simulink model "LF_AC29bus_HVDCdemo_V2_1"  (R2019b)
settings: Solver=FixedStepDiscrete  StartTime=0.0  StopTime=fix(6/Ts)*Ts  FixedStep=Ts  RelTol=1e-3
InitFcn:
  | Ts_avg=150e-6;
  | Ts=50e-6;
  | 
  | %Tc_stab = 1/60/5;
  | %Tc_stab = 2/60;
  | Tc_stab = Ts;
  | 
  | 
  | Ts_avg=150e-6;
  | 
  | Ts=50e-6;
  | 
  | % Rectifier AC side :
  | VLL_nom_R = 735e3; % V
  | Fnom_R = 60;           % Hz
  | 
  | % Inverter AC side :
  | VLL_nom_I = 735e3; % V
  | Fnom_I = 60;           % Hz
  | 
  | % DC :
  | Vdc_nom = 500e3;   % V
  | Idc_nom  = 2000;     % A
undefined symbols (not defined in the file): D1, D11, Delta, test_alpha
libraries: powerlib x223, powerlib_meascontrol x57, simulink x22, sps_avr x7
(part 4 of 10)

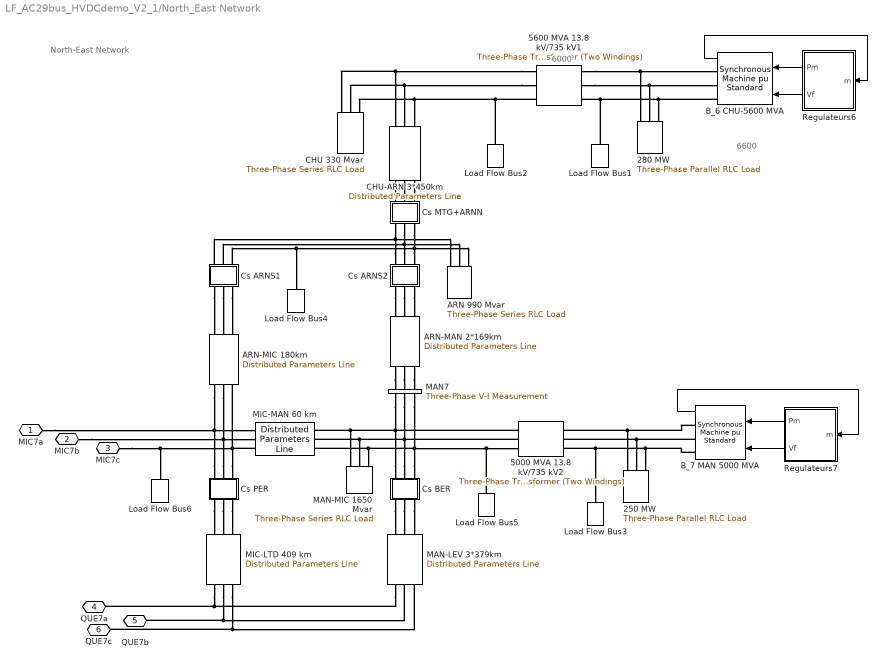
== system LF_AC29bus_HVDCdemo_V2_1/North_East Network ==
  note: 6600
  note: 6000
  note: North-East Network
  250 MW : powerlib/Elements/Three-Phase Parallel RLC Load  LConnTagsString=A|B|C  Configuration=Y (grounded)  NominalVoltage=(13800)*1  Vabc=[1e3 1e3 1e3]  Vabcp=[1e3 1e3 1e3]  NominalFrequency=60  UnbalancedPower=off  ActivePower=250000000  InductivePower=0  CapacitivePower=0  Pabc=[10e3 9e3 11e3]  QLabc=[100 90 110]  QCabc=[100 90 110]  Pabcp=[10e3 9e3 11e3]  QLabcp=[100 90 110]  QCabcp=[100 90 110]  Measurements=None  LoadType=constant PQ
      settings: SourceProductName=Simscape Electrical
  280 MW : powerlib/Elements/Three-Phase Parallel RLC Load  LConnTagsString=A|B|C  Configuration=Y (grounded)  NominalVoltage=(13800)*1  Vabc=[1e3 1e3 1e3]  Vabcp=[1e3 1e3 1e3]  NominalFrequency=60  UnbalancedPower=off  ActivePower=280000000  InductivePower=0  CapacitivePower=0  Pabc=[10e3 9e3 11e3]  QLabc=[100 90 110]  QCabc=[100 90 110]  Pabcp=[10e3 9e3 11e3]  QLabcp=[100 90 110]  QCabcp=[100 90 110]  Measurements=None  LoadType=constant PQ
      settings: SourceProductName=Simscape Electrical
  5000 MVA 13.8 kV/735 kV2 : powerlib/Elements/Three-Phase Transformer (Two Windings)  Winding1Connection=Delta (D1)  Winding2Connection=Yg  CoreType=Three single-phase transformers  SetSaturation=off  Hysteresis=off  DataFile='basic_model'  SetInitialFlux=off  Measurements=None  UNITS=pu  NominalPower=[ 5000e6 60 ]  Winding1="[ 13.8e3 0.002  0.0]"  Winding2=[ 735e3 0.002 0.12]  Rm=500  Lm=500  L0=0.5  Saturation="[ 0,0  ;  0.005,1.2  ;  1.0,1.4 ]"  InitialFluxes=[ 0.8 , -0.8 , 0.7 ]  BreakLoop=off  DiscreteSolver=Trapezoidal iterative  DataType=off  TransfoNumber=0
      settings: SourceProductName=Simscape Electrical
  5600 MVA 13.8 kV/735 kV1 : powerlib/Elements/Three-Phase Transformer (Two Windings)  Winding1Connection=Delta (D1)  Winding2Connection=Yg  CoreType=Three single-phase transformers  SetSaturation=off  Hysteresis=off  DataFile='basic_model'  SetInitialFlux=off  Measurements=None  UNITS=pu  NominalPower=[ 5600e6 60 ]  Winding1="[ 13.8e3 0.002  0.0]"  Winding2=[ 735e3 0.002 0.12]  Rm=500  Lm=500  L0=0.5  Saturation="[ 0,0  ;  0.005,1.2  ;  1.0,1.4 ]"  InitialFluxes=[ 0.8 , -0.8 , 0.7 ]  BreakLoop=off  DiscreteSolver=Trapezoidal iterative  DataType=off  TransfoNumber=0
      settings: SourceProductName=Simscape Electrical
  ARN 990 Mvar : powerlib/Elements/Three-Phase Series RLC Load  LConnTagsString=A|B|C  Configuration=Y (grounded)  NominalVoltage=735e3  Vabc=[1e3 1e3 1e3]  Vabcp=[1e3 1e3 1e3]  NominalFrequency=60  UnbalancedPower=off  ActivePower=3300000  InductivePower=990e6  CapacitivePower=0  Pabc=[10e3 9e3 11e3]  QLabc=[100 90 110]  QCabc=[100 90 110]  Pabcp=[10e3 9e3 11e3]  QLabcp=[100 90 110]  QCabcp=[100 90 110]  Measurements=None  LoadType=constant Z
      settings: SourceProductName=Simscape Electrical
  ARN-MAN 2*169km : powerlib/Elements/Distributed Parameters Line  Phases=3  Frequency=60  Resistance="[0.01273  0.3864]/2"  Inductance="[0.9337e-3  4.1264e-3]/2"  Capacitance=[12.74e-9 7.751e-9]*2  Length=169  x1=[-0.001 1.77895403371725e-09 0 0;-0.00095 1.78335877274119e-09 0 0;-0.0009 1.78712989288485e-09 0 0;-0.00085 1.79026605428719e-09 0 0;-0.0008 1.79276614268501e-09 0 0;-0.00075 1.7946292698088e-09 0 0;-0.0007 1.79585477369837e-09 0 0;-0.00065 1.79644221893802e-09 0 0;-0.0006 1.79639139681125e-09 447147.457758488 -644889.053445503;-0.00055 1.79570232537492e-09 459223.19701965 -636346.501015419;-0.0005 1.79437524945284e-09 471135.776465557 -627577.857703564;-0.00045 1.79241064054876e-09 482880.963613455 -618586.238967152;-0.0004 1.78980919667886e-09 494454.585454275 -609374.839485507;-0.00035 1.78657184212377e-09 505852.529935287 -599946.932025003;-0.0003 1.78269972710015e-09 517070.747421089 -590305.866276268;-0.00025 1.77819422735202e-09 528105.252132427 -580455.067664057;-0.0002 1.773056943662e-09 538952.123562317 -570398.03613021;-0.00015 1.76728970128251e-09 549607.507868989 -560138.344890143;-0.0001 1.76089454928731e-09 560067.619245137 -549679.639163302;-5e-05 1.75387375984347e-09 570328.741262995 -539025.63487803]  x2=[-0.001 3.40571061718068e-09 0 0;-0.00095 3.40987138108151e-09 0 0;-0.0009 3.41282063391716e-09 0 0;-0.00085 3.41455732783211e-09 0 0;-0.0008 3.41508084578731e-09 0 0;-0.00075 3.41439100177931e-09 0 0;-0.0007 3.41248804090641e-09 0 0;-0.00065 3.40937263928153e-09 0 0;-0.0006 3.40504590379205e-09 338825.124939883 -670601.319593136;-0.00055 3.39950937170648e-09 351404.740366806 -664095.897634329;-0.0005 3.39276501012831e-09 363859.503362732 -657354.525565264;-0.00045 3.38481521529709e-09 376184.988809673 -650379.598563337;-0.0004 3.37566281173707e-09 388376.817521339 -643173.5947869;-0.00035 3.36531105125365e-09 400430.657799042 -635739.074494781;-0.0003 3.35376361177806e-09 412342.226970727 -628078.679136641;-0.00025 3.34102459606054e-09 424107.292912585 -620195.130414475;-0.0002 3.32709853021272e-09 435721.675552709 -612091.229315605;-0.00015 3.31199036209949e-09 447181.248356249 -603769.855117503;-0.0001 3.29570545958104e-09 458481.939791554 -595233.9643648;-5e-05 3.27824960860569e-09 469619.734776766 -586486.589818835]  x3=[-0.001 4.69891861565071e-12 0 0;-0.00095 4.9976044278027e-12 0 0;-0.0009 5.29451461489816e-12 0 0;-0.00085 5.58954368616142e-12 0 0;-0.0008 5.88258681916825e-12 0 0;-0.00075 6.17353989708886e-12 0 0;-0.0007 6.46229954568008e-12 0 0;-0.00065 6.74876317001371e-12 0 0;-0.0006 7.03282899092808e-12 1762.60496260231 -1477.81528810955;-0.00055 7.31439608118961e-12 1790.14624540764 -1444.33079403529;-0.0005 7.59336440135186e-12 1817.05149777597 -1410.33313610726;-0.00045 7.869634835299e-12 1843.31116039924 -1375.83439353143;-0.0004 8.14310922546136e-12 1868.91590334437 -1340.84682354679;-0.00035 8.41369040769029e-12 1893.85662936811 -1305.38285707033;-0.0003 8.68128224578015e-12 1918.12447714925 -1269.45509428049;-0.00025 8.94578966562503e-12 1941.71082443704 -1233.07630014032;-0.0002 9.20711868899815e-12 1964.60729111459 -1196.25939986214;-0.00015 9.46517646694184e-12 1986.80574217631 -1159.01747431533;-0.0001 9.71987131275639e-12 2008.29829061826 -1121.36375537869;-5e-05 9.97111273457583e-12 2029.07730024029 -1083.31162123926]  x4=[-0.001 5.93929013944843e-12 0 0;-0.00095 5.74454886917117e-12 0 0;-0.0009 5.54776658803405e-12 0 0;-0.00085 5.34901321184454e-12 0 0;-0.0008 5.14835935673082e-12 0 0;-0.00075 4.94587631405218e-12 0 0;-0.0007 4.74163602506952e-12 0 0;-0.00065 4.53571105538502e-12 0 0;-0.0006 4.32817456915987e-12 2941.48430270319 -8820.70411387501;-0.00055 4.11910030311941e-12 3107.21872626171 -8763.69488470381;-0.0005 3.90856254035483e-12 3271.84916980218 -8703.57195646944;-0.00045 3.69663608393074e-12 3435.31714091192 -8640.35669056202;-0.0004 3.483396230308e-12 3597.56456019916 -8574.07154706452;-0.00035 3.26891874259124e-12 3758.53378192839 -8504.7400767728;-0.0003 3.05327982361058e-12 3918.1676145016 -8432.38691282813;-0.00025 2.83655608884714e-12 4076.4093407782 -8357.03776196514;-0.0002 2.61882453921192e-12 4233.20273822633 -8278.71939537834;-0.00015 2.40016253368777e-12 4388.49209889845 -8197.45963921046;-0.0001 2.18064776184406e-12 4542.22224922416 -8113.28736466595;-5e-05 1.96035821623397e-12 4694.33856961305 -8026.23247775314]  x5=0.000955765248222805  V1=ones(3,3)  V2=ones(3,3)  I1=ones(3,3)  I2=ones(3,3)  nHarmo=1  Measurements=None
      settings: AttributesFormatString=\n  SourceProductName=Simscape Electrical
  ARN-MIC 180km : powerlib/Elements/Distributed Parameters Line  Phases=3  Frequency=60  Resistance="[0.01273  0.3864]"  Inductance="[0.9337e-3  4.1264e-3]"  Capacitance=[12.74e-9 7.751e-9]  Length=180  x1=[-0.00105 1.65528202570484e-09 337720.166187843 -692555.258770577;-0.001 1.65999997031716e-09 350713.785460204 -686066.768257753;-0.00095 1.66412812484431e-09 363582.797794555 -679334.521488954;-0.0009 1.66766502257264e-09 376322.630892093 -672360.910399402;-0.00085 1.67060940685924e-09 388928.758350779 -665148.412679911;-0.0008 1.67296023157838e-09 401396.701273553 -657699.590896577;-0.00075 1.67471666149325e-09 413722.029859663 -650017.091580312;-0.0007 1.67587807255264e-09 425900.364978549 -642103.644286542;-0.00065 1.67644405211275e-09 437927.379725734 -633962.060625409;-0.0006 1.67641439908373e-09 449798.800960145 -625595.233262821;-0.00055 1.67578912400116e-09 461510.410822345 -617006.1348927;-0.0005 1.6745684490223e-09 473058.048233116 -608197.8171808;-0.00045 1.67275280784716e-09 484437.610371872 -599173.40968046;-0.0004 1.6703428455644e-09 495645.054134369 -589936.118720696;-0.00035 1.66733941842215e-09 506676.397569205 -580489.226267001;-0.0003 1.66374359352376e-09 517527.721292583 -570836.088755282;-0.00025 1.6595566484487e-09 528195.169880856 -560980.135899331;-0.0002 1.65478007079863e-09 538674.953240334 -550924.869472268;-0.00015 1.64941555766883e-09 548963.34795389 -540673.862062376;-0.0001 1.64346501504528e-09 559056.698603872 -530230.755803775;-5e-05 1.63693055712744e-09 568951.419070854 -519599.261082393]  x2=[-0.00105 2.20757216589407e-09 202405.879598002 -745458.867777492;-0.001 2.20435426546261e-09 216420.682546405 -741511.432952835;-0.00095 2.20035316845693e-09 230358.592256812 -737300.542646845;-0.0009 2.19557029644773e-09 244214.65665627 -732827.692968796;-0.00085 2.19000734876668e-09 257983.952751074 -728094.47310088;-0.0008 2.18366630190258e-09 271661.588375888 -723102.56473358;-0.00075 2.17654940879921e-09 285242.7039319 -717853.741468168;-0.0007 2.16865919805479e-09 298722.474113422 -712349.868186557;-0.00065 2.15999847302362e-09 312096.109622293 -706592.900388718;-0.0006 2.15057031082007e-09 325358.858869498 -700584.883497896;-0.00055 2.14037806122529e-09 338506.009663382 -694327.952133885;-0.0005 2.12942534549702e-09 351532.890883869 -687824.329354606;-0.00045 2.117716055083e-09 364434.874142089 -681076.325866263;-0.0004 2.10525435023836e-09 377207.375424827 -674086.339202365;-0.00035 2.0920446585475e-09 389845.856723194 -666856.852871891;-0.0003 2.07809167335098e-09 402345.827644964 -659390.435476908;-0.00025 2.06340035207799e-09 414702.847009989 -651689.739799966;-0.0002 2.04797591448504e-09 426912.524428128 -643757.501861571;-0.00015 2.03182384080135e-09 438970.521859132 -635596.539948092;-0.0001 2.01494986978179e-09 450872.555153929 -627209.753610437;-5e-05 1.99735999666791e-09 462614.395576763 -618600.122633857]  x3=[-0.00105 4.80507864505899e-12 25.4663662601597 -574.53320615078;-0.001 4.83653768049388e-12 36.2908676891206 -573.951344402014;-0.00095 4.86627831712063e-12 47.1024751455949 -573.165560473519;-0.0009 4.89428998823267e-12 57.8973473169339 -572.176133550583;-0.00085 4.92056274141663e-12 68.6716488364564 -570.983415171881;-0.0008 4.94508724208841e-12 79.4215516461353 -569.587829104573;-0.00075 4.96785477680969e-12 90.1432363566896 -567.989871193744;-0.0007 4.98885725638379e-12 100.832893604594 -566.19010918623;-0.00065 5.00808721872974e-12 111.486725405528 -564.189182528904;-0.0006 5.02553783153347e-12 122.100946503783 -561.987802141478;-0.00055 5.04120289467534e-12 132.671785717143 -559.586750163923;-0.0005 5.05507684243302e-12 143.195487276771 -556.986879678573;-0.00045 5.06715474545893e-12 153.668312161611 -554.189114407032;-0.0004 5.07743231253163e-12 164.08653942685 -551.19444838198;-0.00035 5.08590589208049e-12 174.446467525947 -548.003945593994;-0.0003 5.09257247348302e-12 184.744415625781 -544.618739613524;-0.00025 5.09742968813462e-12 194.976724914425 -541.040033188136;-0.0002 5.10047581029003e-12 205.139759901111 -537.269097815182;-0.00015 5.10170975767657e-12 215.229909707902 -533.307273290045;-0.0001 5.10113109187859e-12 225.243589352616 -529.155967230113;-5e-05 5.09874001849331e-12 235.177241022557 -524.816654574663]  x4=[-0.00105 7.01566942822821e-13 1335.19730340444 -4937.0942549236;-0.001 6.80396887210245e-13 1428.01688045782 -4911.05082799012;-0.00095 6.58985089823434e-13 1520.32908991326 -4883.262528082;-0.0009 6.37339158172044e-13 1612.10113368227 -4853.73922824988;-0.00085 6.15466782952521e-13 1703.3004055947 -4822.49141798161;-0.0008 5.93375735315632e-13 1793.89450298348 -4789.5301994754;-0.00075 5.71073864105415e-13 1883.8512381972 -4754.86728369523;-0.0007 5.48569093070516e-13 1973.13865003616 -4718.51498621003;-0.00065 5.25869418048926e-13 2061.7250151081 -4680.48622281798;-0.0006 5.02982904127093e-13 2149.57885909932 -4640.79450495766;-0.00055 4.79917682774435e-13 2236.66896795737 -4599.45393490742;-0.0005 4.56681948954273e-13 2322.96439898127 -4556.47920077495;-0.00045 4.33283958212192e-13 2408.43449181528 -4511.88557127866;-0.0004 4.09732023742891e-13 2493.0488793424 -4465.68889032277;-0.00035 3.86034513436542e-13 2576.77749847363 -4417.90557136805;-0.0003 3.62199846905717e-13 2659.59060082928 -4368.5525916002;-0.00025 3.38236492493944e-13 2741.45876330842 -4317.64748589794;-0.0002 3.14152964266941e-13 2822.35289854272 -4265.20834060292;-0.00015 2.89957818987611e-13 2902.24426523115 -4211.25378709378;-0.0001 2.65659653075862e-13 2981.10447835151 -4155.80299516647;-5e-05 2.41267099554346e-13 3058.9055192456 -4098.87566622332]  x5=0.00101797482059234  V1=ones(3,3)  V2=ones(3,3)  I1=ones(3,3)  I2=ones(3,3)  nHarmo=1  Measurements=None
      settings: AttributesFormatString=\n  SourceProductName=Simscape Electrical
  "B_6 CHU-5600 MVA " : powerlib/Machines/Synchronous Machine pu Standard  PresetModel=No  MechanicalLoad=Mechanical power Pm  ShowDetailedParameters=on  RotorType=Salient-pole  Units=per unit standard parameters  MeasurementBus=off  NominalParameters="[ 5600E6  13800   60 ]"  Reactances1=[ 31 32 33 34 35 36 37 ]  Reactances2=[ 1.305, 0.296, 0.252, 0.474, 0.243, 0.18 ]  dAxisTimeConstants=Short-circuit  qAxisTimeConstants=Open-circuit  TimeConstants1=[]  TimeConstants2=[]  TimeConstants3=[]  TimeConstants4=[]  TimeConstants5=[ 1.01, 0.053, 0.1 ]  TimeConstants6=[]  TimeConstants7=[]  TimeConstants8=[]  StatorResistance=2.8544e-3  Mechanical="[ 4.0 0  32]"  PolePairs=32  InitialConditions=[0 -59.3146 0.896045 0.896045 0.896045 11.8671 -108.133 131.867 1.2956]  SetSaturation=off  Saturation=[0.6404,0.7127,0.8441,0.9214,0.9956,1.082,1.19,1.316,1.457;0.7,0.7698,0.8872,0.9466,0.9969,1.046,1.1,1.151,1.201]  LoadFlowParameters=[1 5000000000 0 0 0]  TsPowergui=0  TsBlock=-1  IterativeModel=Trapezoidal non iterative  IterativeDiscreteModel=Trapezoidal non iterative  BusType=PV  Pref=5000000000  Qref=0  Qmin=-Inf  Qmax=Inf  PLF=0  QLF=0
      settings: AttributesFormatString=\n\n  SourceProductName=Simscape Electrical
  B_7 MAN 5000 MVA : powerlib/Machines/Synchronous Machine pu Standard  PresetModel=No  MechanicalLoad=Mechanical power Pm  ShowDetailedParameters=on  RotorType=Salient-pole  Units=per unit standard parameters  MeasurementBus=off  NominalParameters="[ 5000E6  13800   60 ]"  Reactances1=[ 31 32 33 34 35 36 37 ]  Reactances2=[ 1.305, 0.296, 0.252, 0.474, 0.243, 0.18 ]  dAxisTimeConstants=Short-circuit  qAxisTimeConstants=Open-circuit  TimeConstants1=[]  TimeConstants2=[]  TimeConstants3=[]  TimeConstants4=[]  TimeConstants5=[ 1.01, 0.053, 0.1 ]  TimeConstants6=[]  TimeConstants7=[]  TimeConstants8=[]  StatorResistance=2.8544e-3  Mechanical="[ 3.7 0  32]"  PolePairs=32  InitialConditions=[0 -78.7337 0.918283 0.918283 0.918283 -2.27692 -122.277 117.723 1.18952]  SetSaturation=off  Saturation=[0.6404,0.7127,0.8441,0.9214,0.9956,1.082,1.19,1.316,1.457;0.7,0.7698,0.8872,0.9466,0.9969,1.046,1.1,1.151,1.201]  LoadFlowParameters=[1 4500000000 0 0 0]  TsPowergui=0  TsBlock=-1  IterativeModel=Trapezoidal non iterative  IterativeDiscreteModel=Trapezoidal non iterative  BusType=PV  Pref=4500000000  Qref=0  Qmin=-Inf  Qmax=Inf  PLF=0  QLF=0
      settings: AttributesFormatString=\n\n  SourceProductName=Simscape Electrical
  CHU 330 Mvar : powerlib/Elements/Three-Phase Series RLC Load  LConnTagsString=A|B|C  Configuration=Y (grounded)  NominalVoltage=735e3  Vabc=[1e3 1e3 1e3]  Vabcp=[1e3 1e3 1e3]  NominalFrequency=60  UnbalancedPower=off  ActivePower=1100000  InductivePower=330e6  CapacitivePower=0  Pabc=[10e3 9e3 11e3]  QLabc=[100 90 110]  QCabc=[100 90 110]  Pabcp=[10e3 9e3 11e3]  QLabcp=[100 90 110]  QCabcp=[100 90 110]  Measurements=None  LoadType=constant Z
      settings: SourceProductName=Simscape Electrical
  CHU-ARN 3*450km : powerlib/Elements/Distributed Parameters Line  Phases=3  Frequency=60  Resistance="[0.01273  0.3864]/3"  Inductance="[0.9337e-3  4.1264e-3]/3"  Capacitance=[12.74e-9 7.751e-9]*3  Length=450  x1=[-0.00255 -1.47668636008146e-09 70526.907999489 -734521.053767666;-0.0025 -1.43959841142251e-09 84359.0049084098 -733061.266602517;-0.00245 -1.40199898030279e-09 98161.1294645721 -731341.026259902;-0.0024 -1.36390142562115e-09 111928.377838841 -729360.943933024;-0.00235 -1.32531928325737e-09 125655.858593425 -727121.723135704;-0.0023 -1.28626626126292e-09 139338.694419775 -724624.15945243;-0.00225 -1.24675623499054e-09 152972.023871476 -721869.140255687;-0.0022 -1.20680324216445e-09 166551.003091489 -718857.644390675;-0.00215 -1.16642147789276e-09 180070.807533156 -715590.741827537;-0.0021 -1.12562528962402e-09 193526.633674335 -712069.593281197;-0.00205 -1.08442917204968e-09 206913.70072407 -708295.449798968;-0.002 -1.04284776195414e-09 220227.252321181 -704269.652316058;-0.00195 -1.00089583301443e-09 233462.558224181 -699993.631179143;-0.0019 -9.58588290551127e-10 246614.915991903 -695468.905638173;-0.00185 -9.15940166232625e-10 259679.652654259 -690697.083306586;-0.0018 -8.72966612734418e-10 272652.126372523 -685679.859590136;-0.00175 -8.29682898355439e-10 285527.728088551 -680419.01708452;-0.0017 -7.86104401593308e-10 298301.883162364 -674916.424942028;-0.00165 -7.4224660568042e-10 310970.052997488 -669174.038207449;-0.0016 -6.98125093082829e-10 323527.736653504 -663193.897123447;-0.00155 -6.53755539963869e-10 335970.472445202 -656978.126405672;-0.0015 -6.09153710614495e-10 348293.839527803 -650528.934487864;-0.00145 -5.64335451852297e-10 360493.459467662 -643848.612737203;-0.0014 -5.19316687391205e-10 372564.997797904 -636939.534640197;-0.00135 -4.74113412183872e-10 384504.165558441 -629804.154959397;-0.0013 -4.28741686738736e-10 396306.720819817 -622445.008861226;-0.00125 -3.83217631413806e-10 407968.470190347 -614864.711015252;-0.0012 -3.37557420689171e-10 419485.270306009 -607065.954665206;-0.00115 -2.91777277420284e-10 430853.029302559 -599051.510672083;-0.0011 -2.45893467074062e-10 442067.708269356 -590824.226529673;-0.00105 -1.99922291949839e-10 453125.322684362 -582387.025352856;-0.001 -1.53880085387241e-10 464021.943829828 -573742.904839035;-0.00095 -1.07783205963022e-10 474753.700188146 -564894.93620307;-0.0009 -6.1648031678947e-11 485316.778817384 -555846.263086086;-0.00085 -1.54909541427609e-11 495707.426706 -546600.100438555;-0.0008 3.067162725567e-11 505921.952106278 -537159.73337804;-0.00075 7.68233111709838e-11 515956.725845979 -527528.516022004;-0.0007 1.22947700129642e-10 525808.182617776 -517709.870296115;-0.00065 1.69028406355873e-10 535472.822245987 -507707.284718447;-0.0006 2.15049057594176e-10 544947.210930171 -497524.313160026;-0.00055 2.60993302926296e-10 554227.982465141 -487164.57358216;-0.0005 3.06844818580638e-10 563311.839436964 -476631.746750992;-0.00045 3.52587313732015e-10 572195.554394511 -465929.574929742;-0.0004 3.98204536289709e-10 580875.970996158 -455061.860549098;-0.00035 4.43680278671758e-10 589350.005131219 -444032.464856231;-0.0003 4.88998383563431e-10 597614.646015717 -432845.306542914;-0.00025 5.34142749657847e-10 605666.957262098 -421504.360353226;-0.0002 5.79097337376693e-10 613504.077922519 -410013.655671348;-0.00015 6.2384617456901e-10 621123.223505326 -398377.275089938;-0.0001 6.68373362186019e-10 628521.686964373 -386599.352959609;-5e-05 7.12663079929983e-10 635696.839660821 -374684.073920012]  x2=[-0.00255 1.63896785414151e-09 -245055.631636569 -719265.627917785;-0.0025 1.65992719155378e-09 -231455.029793756 -723756.779042432;-0.00245 1.68029676473884e-09 -217772.193080958 -727990.782829739;-0.0024 1.70006933648431e-09 -204011.982944907 -731966.13495832;-0.00235 1.71923788168961e-09 -190179.288322742 -735681.423004494;-0.0023 1.7377955898619e-09 -176279.023904997 -739135.326944109;-0.00225 1.75573586753583e-09 -162316.128389432 -742326.61962154;-0.0022 1.77305234061617e-09 -148295.562726338 -745254.167185695;-0.00215 1.78973885664249e-09 -134222.308355934 -747916.929492865;-0.0021 1.80578948697509e-09 -120101.365438486 -750313.960476281;-0.00205 1.82119852890146e-09 -105937.751077775 -752444.408482248;-0.002 1.83596050766235e-09 -91736.4975385414 -754307.516572735;-0.00195 1.85007017839702e-09 -77502.6504585462 -755902.622794307;-0.0019 1.86352252800663e-09 -63241.2670558813 -757229.16041332;-0.00185 1.87631277693542e-09 -48957.4143321619 -758286.658117274;-0.0018 1.88843638086885e-09 -34656.1672722469 -759074.740182271;-0.00175 1.89988903234816e-09 -20342.6070411195 -759593.126606505;-0.0017 1.91066666230084e-09 -6021.81917857414 -759841.633209747;-0.00165 1.92076544148626e-09 8301.10820765171 -759820.171698786;-0.0016 1.93018178185627e-09 22621.086249658 -759528.749698794;-0.00155 1.93891233782998e-09 36933.0271274329 -758967.47075062;-0.0015 1.94695400748241e-09 51231.8458765305 -758136.534274001;-0.00145 1.95430393364664e-09 65512.4621947345 -757036.235496711;-0.0014 1.9609595049289e-09 79769.8022470661 -755666.965349666;-0.00135 1.96691835663639e-09 93998.8004684927 -754029.210328031;-0.0013 1.97217837161748e-09 108194.401363699 -752123.552318364;-0.00125 1.9767376810139e-09 122351.561303281 -749950.668391884;-0.0012 1.98059466492472e-09 136465.250315724 -747511.330563903;-0.00115 1.98374795298193e-09 150530.453874525 -744806.405519537;-0.0011 1.9861964248373e-09 164542.174679833 -741836.854305772;-0.00105 1.98793921056043e-09 178495.434433964 -738603.731990017;-0.001 1.98897569094786e-09 192385.275610168 -735108.187285234;-0.00095 1.98930549774303e-09 206206.763214012 -731351.462141813;-0.0009 1.98892851376717e-09 219954.986536765 -727334.89130631;-0.00085 1.98784487296088e-09 233625.060900142 -723059.901847216;-0.0008 1.98605496033659e-09 247212.129391815 -718528.012647931;-0.00075 1.98355941184173e-09 260711.364591045 -713740.833867109;-0.0007 1.98035911413279e-09 274117.970283844 -708700.066366574;-0.00065 1.97645520426032e-09 287427.183167046 -703407.501107019;-0.0006 1.97184906926489e-09 300634.274540687 -697865.018511678;-0.00055 1.96654234568435e-09 313734.551988089 -692074.587798226;-0.0005 1.96053691897231e-09 326723.361043055 -686038.266279124;-0.00045 1.95383492282829e-09 339596.086843573 -679758.198630666;-0.0004 1.9464387384396e-09 352348.155771463 -673236.616130983;-0.00035 1.93835099363534e-09 364975.037077354 -666475.835867285;-0.0003 1.92957456195273e-09 377472.244490443 -659478.259912606;-0.00025 1.92011256161616e-09 389835.337812444 -652246.374472364;-0.0002 1.90996835442928e-09 402059.924495167 -644782.749001019;-0.00015 1.89914554458062e-09 414141.661201173 -637090.035289164;-0.0001 1.88764797736297e-09 426076.255346938 -629170.96652135;-5e-05 1.87547973780723e-09 437859.466627991 -621028.356305003]  x3=[-0.00255 -3.61445126531467e-12 -1564.23608055638 -1972.57753493018;-0.0025 -3.33430168268211e-12 -1526.77778904953 -2001.71090545922;-0.00245 -3.05296743853838e-12 -1488.77704066415 -2030.13307763493;-0.0024 -2.77054848960079e-12 -1450.24733688522 -2057.83395319487;-0.00235 -2.48714517797714e-12 -1411.20236713302 -2084.80369014987;-0.0023 -2.2028581955146e-12 -1371.65600389938 -2111.03270628079;-0.00225 -1.91778854802435e-12 -1331.62229781886 -2136.5116825431;-0.0022 -1.63203751939477e-12 -1291.1154726766 -2161.23156637786;-0.00215 -1.34570663560569e-12 -1250.1499203547 -2185.18357492804;-0.0021 -1.05889762865672e-12 -1208.74019571883 -2208.35919815906;-0.00205 -7.71712400422351e-13 -1166.90101144698 -2230.75020188234;-0.002 -4.84252986446714e-13 -1124.6472328021 -2252.34863068086;-0.00195 -1.96621519690819e-13 -1081.99387235055 -2273.14681073573;-0.0019 9.10798057547839e-14 -1038.95608462819 -2293.13735255261;-0.00185 3.7874877097909e-13 -995.549160756075 -2312.31315358716;-0.0018 6.66283168568525e-13 -951.788523007569 -2330.6674007686;-0.00175 9.53580838920754e-13 -907.689719328891 -2348.19357292029;-0.0017 1.2405397065415e-12 -863.268417815008 -2364.88544307673;-0.00165 1.52705781631149e-12 -818.54040114283 -2380.73708069592;-0.0016 1.81303336971061e-12 -773.521560963703 -2395.7428537665;-0.00155 2.09836476098644e-12 -728.227892257179 -2409.89743080875;-0.0015 2.38295061325431e-12 -682.675487648079 -2423.19578276885;-0.00145 2.66668981451599e-12 -636.880531688857 -2435.63318480565;-0.0014 2.94948155358433e-12 -590.859295109309 -2447.20521796946;-0.00135 3.23122535590099e-12 -544.628129035654 -2457.90777077197;-0.0013 3.51182111923455e-12 -498.203459181065 -2467.73704064715;-0.00125 3.7911691492464e-12 -451.601780009682 -2476.68953530221;-0.0012 4.06917019491163e-12 -404.839648876218 -2484.76207395842;-0.00115 4.34572548378243e-12 -357.933680143199 -2491.95178848124;-0.0011 4.62073675708153e-12 -310.90053927797 -2498.25612439934;-0.00105 4.89410630461303e-12 -263.756936931524 -2503.67284181218;-0.001 5.16573699947836e-12 -216.519623001296 -2508.20001618586;-0.00095 5.43553233258504e-12 -169.20538068 -2511.83603903688;-0.0009 5.70339644693588e-12 -121.831020492639 -2514.57961850363;-0.00085 5.96923417168653e-12 -74.4133743238106 -2516.4297798054;-0.0008 6.23295105595918e-12 -26.9692894374127 -2517.38586558867;-0.00075 6.49445340240059e-12 20.4843775091049 -2517.44753616074;-0.0007 6.75364830047222e-12 67.9307664538323 -2516.61476961033;-0.00065 7.010443659461e-12 115.353019920699 -2514.88786181543;-0.0006 7.26474824119862e-12 162.734289008855 -2512.26742633817;-0.00055 7.5164716924781e-12 210.057739379005 -2508.75439420679;-0.0005 7.76552457715581e-12 257.306557234568 -2504.35001358488;-0.00045 8.01181840792772e-12 304.463955295541 -2499.05584932789;-0.0004 8.25526567776851e-12 351.513178762938 -2492.8737824272;-0.00035 8.49577989102241e-12 398.437511271693 -2485.80600934171;-0.0003 8.73327559413469e-12 445.2202808299 -2477.85504121757;-0.00025 8.9676684060129e-12 491.844865742297 -2469.02370299588;-0.0002 9.19887504800706e-12 538.294700515873 -2459.31513240907;-0.00015 9.42681337349819e-12 584.55328174551 -2448.73277886602;-0.0001 9.6514023970846e-12 630.604173977562 -2437.28040222658;-5e-05 9.87256232335563e-12 676.431015549296 -2424.96207146563]  x4=[-0.00255 -3.6279512546673e-12 -5139.72013674173 -13300.2137364959;-0.0025 -3.76512484764398e-12 -4888.11818610537 -13394.7263740201;-0.00245 -3.90096070969037e-12 -4634.77951035283 -13484.4799290442;-0.0024 -4.0354105789715e-12 -4379.79411950932 -13569.4425125574;-0.00235 -4.168426686089e-12 -4123.25260867006 -13649.5839377585;-0.0023 -4.2999617710534e-12 -3865.24612581228 -13724.8757307806;-0.00225 -4.42996910007531e-12 -3605.86633941084 -13795.2911408081;-0.0022 -4.55840248216978e-12 -3345.20540586875 -13860.8051495812;-0.00215 -4.68521628556771e-12 -3083.35593677455 -13921.3944802845;-0.0021 -4.81036545392859e-12 -2820.41096599778 -13977.0376058174;-0.00205 -4.93380552234882e-12 -2556.46391663451 -14027.7147564422;-0.002 -5.05549263315985e-12 -2291.60856781457 -14073.4079268087;-0.00195 -5.17538355151064e-12 -2025.93902138224 -14114.1008823509;-0.0019 -5.29343568072878e-12 -1759.54966846237 -14149.7791650556;-0.00185 -5.40960707745487e-12 -1492.53515592359 -14180.4300985989;-0.0018 -5.52385646654483e-12 -1224.9903527508 -14206.0427928498;-0.00175 -5.63614325573472e-12 -957.01031633861 -14226.6081477403;-0.0017 -5.74642755006301e-12 -688.690258717943 -14242.1188564975;-0.00165 -5.85467016604505e-12 -420.125512727634 -14252.5694082405;-0.0016 -5.9608326455948e-12 -151.411498143132 -14257.9560899381;-0.00155 -6.06487726968878e-12 117.3563122257 -14258.2769877278;-0.0015 -6.16676707176747e-12 386.082426455604 -14253.5319875963;-0.00145 -6.26646585086935e-12 654.671367437766 -14243.7227754195;-0.0014 -6.36393818449293e-12 923.02770680037 -14228.8528363637;-0.00135 -6.4591494411822e-12 1191.05609881385 -14208.9274536476;-0.0013 -6.55206579283103e-12 1458.66131426678 -14183.9537066646;-0.00125 -6.64265422670209e-12 1725.74827430034 -14153.9404684682;-0.0012 -6.73088255715619e-12 1992.2220841894 -14118.8984026191;-0.00115 -6.81671943708763e-12 2257.98806705814 -14078.8399593962;-0.0011 -6.90013436906168e-12 2522.95179751833 -14033.7793713739;-0.00105 -6.9810977161502e-12 2787.0191352182 -13983.7326483644;-0.001 -7.0595807124615e-12 3050.09625829004 -13928.7175717302;-0.00095 -7.13555547336069e-12 3312.08969668471 -13868.7536880659;-0.0009 -7.20899500537699e-12 3572.90636538105 -13803.862302254;-0.00085 -7.27987321579435e-12 3832.45359745859 -13734.0664698948;-0.0008 -7.34816492192212e-12 4090.63917702163 -13659.3909891153;-0.00075 -7.41384586004228e-12 4347.37137196314 -13579.8623917581;-0.0007 -7.47689269403027e-12 4602.5589665567 -13495.5089339552;-0.00065 -7.53728302364618e-12 4856.11129386508 -13406.3605860886;-0.0006 -7.59499539249345e-12 5107.9382679537 -13312.4490221417;-0.00055 -7.65000929564224e-12 5357.95041589776 -13213.807608446;-0.0005 -7.7023051869147e-12 5606.05890957157 -13110.4713918261;-0.00045 -7.7518644858297e-12 5852.17559720872 -13002.4770871478;-0.0004 -7.79866958420429e-12 6096.213034722 -12889.8630642733;-0.00035 -7.8427038524099e-12 6338.08451677189 -12772.6693344286;-0.0003 -7.88395164528071e-12 6577.7041075725 -12650.9375359879;-0.00025 -7.92239830767231e-12 6814.98667142421 -12524.7109196797;-0.0002 -7.95803017966864e-12 7049.84790296192 -12394.0343332196;-0.00015 -7.99083460143523e-12 7282.2043571084 -12258.9542053765;-0.0001 -8.02079991771723e-12 7511.97347872187 -12119.5185294768;-5e-05 -8.04791548198045e-12 7739.07363192749 -11975.776846352]  x5=0.00254493705148084  V1=ones(3,3)  V2=ones(3,3)  I1=ones(3,3)  I2=ones(3,3)  nHarmo=1  Measurements=None
      settings: AttributesFormatString=\n  SourceProductName=Simscape Electrical
  "Cs ARNS1 " : Subsystem  mask{Xc=25}
      mask prompts: Xc "Condensator Reactance at  60Hz  (ohm):"
      mask help: Series Compensation
      mask init:
      | Cs=1/Xc/(2*pi*60);
      mask Display: disp('Cs')
  Cs ARNS2 : Subsystem  mask{Xc=25/2}
      mask prompts: Xc "Condensator Reactance at  60Hz  (ohm):"
      mask help: Series Compensation
      mask init:
      | Cs=1/Xc/(2*pi*60);
      mask Display: disp('Cs')
  Cs BER : Subsystem  mask{Xc=22/3}
      mask prompts: Xc "Condensator Reactance at  60Hz  (ohm):"
      mask help: Series Compensation
      mask init:
      | Cs=1/Xc/(2*pi*60);
      mask Display: disp('Cs')
  "Cs MTG+ARNN " : Subsystem  mask{Xc=(30+25)/3}
      mask prompts: Xc "Condensator Reactance at  60Hz  (ohm):"
      mask help: Series Compensation
      mask init:
      | Cs=1/Xc/(2*pi*60);
      mask Display: disp('Cs')
  "Cs PER " : Subsystem  mask{Xc=22}
      mask prompts: Xc "Condensator Reactance at  60Hz  (ohm):"
      mask help: Series Compensation
      mask init:
      | Cs=1/Xc/(2*pi*60);
      mask Display: disp('Cs')
  Load Flow Bus1 : powerlib/Measurements/Load Flow Bus  LConnTagsString=a  Phases=single  Connectors=on one side  ID=CHU_13.8  Vbase=13.8e3  Vref=1  Vangle=0  VLF=1  VLFb=1  VLFc=1  angleLF=7.032  angleLFb=0  angleLFc=0
      settings: AttributesFormatString=%<ID>\n%<Vbase>V\n%<VLF>pu\n%<angleLF>deg.  SourceProductName=Simscape Electrical
  Load Flow Bus2 : powerlib/Measurements/Load Flow Bus  LConnTagsString=a  Phases=single  Connectors=on one side  ID=CHU7  Vbase=735e3  Vref=1  Vangle=0  VLF=1.011  VLFb=1  VLFc=1  angleLF=31.29  angleLFb=0  angleLFc=0
      settings: AttributesFormatString=%<ID>\n%<Vbase>V\n%<VLF>pu\n%<angleLF>deg.  SourceProductName=Simscape Electrical
  Load Flow Bus3 : powerlib/Measurements/Load Flow Bus  LConnTagsString=a  Phases=single  Connectors=on one side  ID=MAN_13.8  Vbase=13.8e3  Vref=1  Vangle=0  VLF=1  VLFb=1  VLFc=1  angleLF=-13.73  angleLFb=0  angleLFc=0
      settings: AttributesFormatString=%<ID>\n%<Vbase>V\n%<VLF>pu\n%<angleLF>deg.  SourceProductName=Simscape Electrical
  Load Flow Bus4 : powerlib/Measurements/Load Flow Bus  LConnTagsString=a  Phases=single  Connectors=on one side  ID=ARN7  Vbase=735e3  Vref=1  Vangle=0  VLF=1.062  VLFb=1  VLFc=1  angleLF=15.17  angleLFb=0  angleLFc=0
      settings: AttributesFormatString=%<ID>\n%<Vbase>V\n%<VLF>pu\n%<angleLF>deg.  SourceProductName=Simscape Electrical
  Load Flow Bus5 : powerlib/Measurements/Load Flow Bus  LConnTagsString=a  Phases=single  Connectors=on one side  ID=MAN7  Vbase=735e3  Vref=1  Vangle=0  VLF=1.024  VLFb=1  VLFc=1  angleLF=10.53  angleLFb=0  angleLFc=0
      settings: AttributesFormatString=%<ID>\n%<Vbase>V\n%<VLF>pu\n%<angleLF>deg.  SourceProductName=Simscape Electrical
  Load Flow Bus6 : powerlib/Measurements/Load Flow Bus  LConnTagsString=a  Phases=single  Connectors=on one side  ID=MIC7  Vbase=735e3  Vref=1  Vangle=0  VLF=1.051  VLFb=1  VLFc=1  angleLF=8.512  angleLFb=0  angleLFc=0
      settings: AttributesFormatString=%<ID>\n%<Vbase>V\n%<VLF>pu\n%<angleLF>deg.  SourceProductName=Simscape Electrical
  MAN-LEV 3*379km : powerlib/Elements/Distributed Parameters Line  Phases=3  Frequency=60  Resistance="[0.01273  0.3864]/3"  Inductance="[0.9337e-3  4.1264e-3]/3"  Capacitance=[12.74e-9 7.751e-9]*3  Length=379  x1=[-0.00215 2.69555694980098e-09 0 0;-0.0021 2.73457468859354e-09 0 0;-0.00205 2.77262084602024e-09 0 0;-0.002 2.80968190446251e-09 0 0;-0.00195 2.84574469630276e-09 0 0;-0.0019 2.88079640860276e-09 0 0;-0.00185 2.91482458765603e-09 0 0;-0.0018 2.9478171434126e-09 0 0;-0.00175 2.97976235377449e-09 0 0;-0.0017 3.01064886876057e-09 0 0;-0.00165 3.04046571453914e-09 0 0;-0.0016 3.06920229732687e-09 0 0;-0.00155 3.09684840715273e-09 0 0;-0.0015 3.12339422148554e-09 0 0;-0.00145 3.14883030872386e-09 0 0;-0.0014 3.17314763154703e-09 0 0;-0.00135 3.19633755012602e-09 194395.779276237 -715238.323898765;-0.0013 3.21839182519319e-09 207842.400313668 -711447.235906672;-0.00125 3.23930262096962e-09 221215.175935933 -707403.374099303;-0.0012 3.25906250794914e-09 234509.354859531 -703108.1752415;-0.00115 3.277664465538e-09 247720.21372599 -698563.165396967;-0.0011 3.29510188454924e-09 260843.058780062 -693769.959386059;-0.00105 3.31136856955091e-09 273873.227537385 -688730.260212049;-0.001 3.3264587410673e-09 286806.090441043 -683445.858456055;-0.00095 3.34036703763231e-09 299637.052506429 -677918.631640861;-0.0009 3.3530885176944e-09 312361.554953816 -672150.543563834;-0.00085 3.36461866137228e-09 324975.076828074 -666143.643599203;-0.0008 3.37495337206081e-09 337473.136604943 -659900.065969923;-0.00075 3.38408897788648e-09 349851.293783294 -653422.028989395;-0.0007 3.39202223301204e-09 362105.150462822 -646711.834273314;-0.00065 3.39875031878974e-09 374230.352906597 -639771.865921911;-0.0006 3.40427084476271e-09 386222.593087927 -632604.589672894;-0.00055 3.40858184951438e-09 398077.610220976 -625212.552025388;-0.0005 3.41168180136528e-09 409791.192274608 -617598.379335171;-0.00045 3.41356959891729e-09 421359.177468894 -609764.776881544;-0.0004 3.41424457144491e-09 432777.455753776 -601714.527906157;-0.00035 3.41370647913362e-09 444041.97026935 -593450.49262414;-0.0003 3.41195551316507e-09 455148.718787246 -584975.607207879;-0.00025 3.40899229564911e-09 466093.7551326 -576292.882743807;-0.0002 3.40481787940284e-09 476873.190586117 -567405.404162582;-0.00015 3.39943374757645e-09 487483.195265706 -558316.329143027;-0.0001 3.39284181312635e-09 497919.999487227 -549028.886990216;-5e-05 3.38504441813547e-09 508179.895103834 -539546.377488123]  x2=[-0.00215 1.92253672127361e-09 0 0;-0.0021 1.85442757786035e-09 0 0;-0.00205 1.78565956515875e-09 0 0;-0.002 1.71625711611628e-09 0 0;-0.00195 1.64624488909261e-09 0 0;-0.0019 1.57564775909864e-09 0 0;-0.00185 1.50449080895849e-09 0 0;-0.0018 1.43279932039773e-09 0 0;-0.00175 1.36059876506087e-09 0 0;-0.0017 1.28791479546144e-09 0 0;-0.00165 1.21477323586775e-09 0 0;-0.0016 1.14120007312763e-09 0 0;-0.00155 1.06722144743549e-09 0 0;-0.0015 9.92863643044777e-10 0 0;-0.00145 9.18153078929328e-10 0 0;-0.0014 8.4311629939683e-10 0 0;-0.00135 7.67779964657754e-10 -157064.651836757 -753550.814995821;-0.0013 6.9217084135311e-10 -142833.476838404 -756377.385326958;-0.00125 6.16315793044386e-10 -128551.553785848 -758935.218374669;-0.0012 5.40241770669054e-10 -114223.956978345 -761223.405353051;-0.00115 4.63975802965028e-10 -99855.7769428187 -763241.133280166;-0.0011 3.87544986867484e-10 -85452.1186252198 -764987.68526689;-0.00105 3.10976477881448e-10 -71018.0995767636 -766462.440771617;-0.001 2.34297480433571e-10 -56558.8481356889 -767664.875820739;-0.00095 1.57535238206532e-10 -42079.5016051833 -768594.56319481;-0.0009 8.07170244594799e-11 -27585.2044281237 -769251.172580331;-0.00085 3.8701323379814e-12 -13081.1063592811 -769634.470687114;-0.0008 -7.29781348231086e-11 1427.63936436365 -769744.321331168;-0.00075 -1.4980047320039e-10 15935.8778545402 -769580.685483081;-0.0007 -2.26569588182836e-10 30438.4544031956 -769143.621281891;-0.00065 -3.03258204069439e-10 44930.2163139378 -768433.284014428;-0.0006 -3.79839073760135e-10 59406.0147327642 -767449.92606014;-0.00055 -4.56284988436573e-10 73860.7064774248 -766193.896801427;-0.0005 -5.32568787229274e-10 88289.1558647705 -764665.642499502;-0.00045 -6.08663366867762e-10 102686.236535437 -762865.706135843;-0.0004 -6.84541691310224e-10 117046.833275214 -760794.72721927;-0.00035 -7.6017680134929e-10 131365.843832462 -758453.441558729;-0.0003 -8.35541824190508e-10 145638.180730909 -755842.681001868;-0.00025 -9.10609983000122e-10 159858.773077217 -752963.373139481;-0.0002 -9.85354606418753e-10 174022.568362636 -749816.540975942;-0.00015 -1.05974913803761e-09 188124.534258145 -746403.302565733;-0.0001 -1.13376714583383e-09 202159.66040241 -742724.870616211;-5e-05 -1.20738233156171e-09 216122.96018194 -738782.552056731]  x3=[-0.00215 3.09797485655976e-11 0 0;-0.0021 3.09765861063957e-11 0 0;-0.00205 3.09624178136488e-11 0 0;-0.002 3.09372487212839e-11 0 0;-0.00195 3.09010877717598e-11 0 0;-0.0019 3.08539478128895e-11 0 0;-0.00185 3.0795845593276e-11 0 0;-0.0018 3.07268017563612e-11 0 0;-0.00175 3.06468408330917e-11 0 0;-0.0017 3.05559912332028e-11 0 0;-0.00165 3.04542852351247e-11 0 0;-0.0016 3.03417589745142e-11 0 0;-0.00155 3.02184524314159e-11 0 0;-0.0015 3.00844094160575e-11 0 0;-0.00145 2.9939677553284e-11 0 0;-0.0014 2.97843082656371e-11 0 0;-0.00135 2.9618356755085e-11 -1018.65488165677 -236.511496511394;-0.0013 2.9441881983409e-11 -1014.01604188363 -255.670064207239;-0.00125 2.92549466512554e-11 -1009.01692703917 -274.737793546675;-0.0012 2.90576171758575e-11 -1003.65931328508 -293.707909856259;-0.00115 2.88499636674382e-11 -997.945104156024 -312.573673143997;-0.0011 2.86320599043004e-11 -991.876329883296 -331.328380494023;-0.00105 2.84039833066136e-11 -985.455146673496 -349.965368448119;-0.001 2.81658149089068e-11 -978.683835942444 -368.478015373206;-0.00095 2.79176393312777e-11 -971.5648035046 -386.859743813983;-0.0009 2.76595447493274e-11 -964.100578718292 -405.104022829861;-0.00085 2.73916228628318e-11 -956.293813587044 -423.204370315378;-0.0008 2.71139688631615e-11 -948.147281817334 -441.15435530326;-0.00075 2.68266813994605e-11 -939.66387783311 -458.947600249311;-0.0007 2.65298625435967e-11 -930.846615747412 -476.577783298327;-0.00065 2.62236177538962e-11 -921.698628291475 -494.038640530218;-0.0006 2.59080558376746e-11 -912.223165701682 -511.323968185552;-0.00055 2.55832889125781e-11 -902.423594564775 -528.427624869719;-0.0005 2.52494323667488e-11 -892.303396621714 -545.34353373494;-0.00045 2.49066048178278e-11 -881.866167530642 -562.065684639343;-0.0004 2.45549280708108e-11 -871.115615589357 -578.588136282336;-0.00035 2.41945270747714e-11 -860.055560417772 -594.905018315523;-0.0003 2.38255298784674e-11 -848.689931600827 -611.010533428414;-0.00025 2.34480675848456e-11 -837.022767292321 -626.898959408175;-0.0002 2.30622743044618e-11 -825.058212780179 -642.564651172713;-0.00015 2.26682871078312e-11 -812.800519013648 -658.002042776336;-0.0001 2.2266245976729e-11 -800.254041092958 -673.205649387315;-5e-05 2.18562937544546e-11 -787.423236721971 -688.170069236616]  x4=[-0.00215 -1.8010968641509e-11 0 0;-0.0021 -1.80272695994267e-11 0 0;-0.00205 -1.80371655542948e-11 0 0;-0.002 -1.80406529901275e-11 0 0;-0.00195 -1.80377306678555e-11 0 0;-0.0019 -1.8028399625766e-11 0 0;-0.00185 -1.80126631791338e-11 0 0;-0.0018 -1.79905269190435e-11 0 0;-0.00175 -1.79619987104029e-11 0 0;-0.0017 -1.79270886891486e-11 0 0;-0.00165 -1.7885809258645e-11 0 0;-0.0016 -1.78381750852773e-11 0 0;-0.00155 -1.77842030932403e-11 0 0;-0.0015 -1.77239124585258e-11 0 0;-0.00145 -1.76573246021094e-11 0 0;-0.0014 -1.75844631823392e-11 0 0;-0.00135 -1.75053540865309e-11 -2630.54986023999 -15922.6329346055;-0.0013 -1.74200254217694e-11 -2329.96516568655 -15969.3858938231;-0.00125 -1.73285075049231e-11 -2028.55264560415 -16010.4650062728;-0.0012 -1.7230832851872e-11 -1726.41939042597 -16045.8556767415;-0.00115 -1.71270361659553e-11 -1423.67274665891 -16075.5453310924;-0.0011 -1.70171543256413e-11 -1120.42027874395 -16099.5234207328;-0.00105 -1.69012263714245e-11 -816.769730838967 -16117.7814263616;-0.001 -1.67792934919551e-11 -512.828988537762 -16130.3128609964;-0.00095 -1.66513990094046e-11 -208.706040538826 -16137.113272278;-0.0009 -1.65175883640737e-11 95.4910597225371 -16138.1802440527;-0.00085 -1.63779090982475e-11 399.654232465072 -16133.5133972306;-0.0008 -1.62324108393041e-11 703.675409961811 -16123.1143899201;-0.00075 -1.60811452820819e-11 1007.44657493603 -16106.9869168389;-0.0007 -1.59241661705133e-11 1310.85979893924 -16085.1367080015;-0.00065 -1.57615292785291e-11 1613.80728069771 -16057.5715266831;-0.0006 -1.55932923902427e-11 1916.18138441368 -16024.3011666612;-0.00055 -1.54195152794193e-11 2217.87467800789 -15985.3374487364;-0.0005 -1.52402596882389e-11 2518.77997128967 -15940.6942165322;-0.00045 -1.50555893053596e-11 2818.79035404113 -15890.3873315763;-0.0004 -1.48655697432891e-11 3117.79923400179 -15834.4346676654;-0.00035 -1.4670268515073e-11 3415.70037474039 -15772.8561045147;-0.0003 -1.44697550103076e-11 3712.3879334001 -15705.6735206943;-0.00025 -1.42641004704866e-11 4007.75649830404 -15632.9107858565;-0.0002 -1.40533779636886e-11 4301.70112640755 -15554.5937522544;-0.00015 -1.38376623586169e-11 4594.1173805839 -15470.7502455572;-0.0001 -1.36170302979988e-11 4884.90136673036 -15381.4100549635;-5e-05 -1.3391560171355e-11 5173.94977068125 -15286.6049226177]  x5=0.00214340253891386  V1=ones(3,3)  V2=ones(3,3)  I1=ones(3,3)  I2=ones(3,3)  nHarmo=1  Measurements=None
      settings: AttributesFormatString=\n  SourceProductName=Simscape Electrical
  MAN-MIC 1650 Mvar : powerlib/Elements/Three-Phase Series RLC Load  LConnTagsString=A|B|C  Configuration=Y (grounded)  NominalVoltage=735e3  Vabc=[1e3 1e3 1e3]  Vabcp=[1e3 1e3 1e3]  NominalFrequency=60  UnbalancedPower=off  ActivePower=5500000  InductivePower=1650e6  CapacitivePower=0  Pabc=[10e3 9e3 11e3]  QLabc=[100 90 110]  QCabc=[100 90 110]  Pabcp=[10e3 9e3 11e3]  QLabcp=[100 90 110]  QCabcp=[100 90 110]  Measurements=None  LoadType=constant Z
      settings: SourceProductName=Simscape Electrical
  MAN7 : powerlib/Measurements/Three-Phase V-I Measurement  VoltageMeasurement=no  SetLabelV=on  LabelV=Vabc_MAN7  Vpu=on  VpuLL=off  CurrentMeasurement=no  SetLabelI=on  LabelI=Iabc_MAN7  Ipu=on  Pbase=100e6  Vbase=735e3  OutputType=Magnitude  PhasorSimulation=off  PSBequivalent=0
      settings: SourceProductName=Simscape Electrical
  MIC-LTD 409 km : powerlib/Elements/Distributed Parameters Line  Phases=3  Frequency=60  Resistance="[0.01273  0.3864]"  Inductance="[0.9337e-3  4.1264e-3]"  Capacitance=[12.74e-9 7.751e-9]  Length=409  x1=[-0.00235 2.28352820606062e-09 -120542.623914577 -752200.690894203;-0.0023 2.29896500098363e-09 -106343.364281404 -754339.120639806;-0.00225 2.3135849845886e-09 -92106.321357268 -756209.537287721;-0.0022 2.32738296246494e-09 -77836.5534957289 -757811.276287818;-0.00215 2.34035403225683e-09 -63539.1306773609 -759143.768549858;-0.0021 2.35249358540493e-09 -49219.1327084123 -760206.540645685;-0.00205 2.36379730878382e-09 -34881.647415975 -760999.214977433;-0.002 2.37426118623439e-09 -20531.768840304 -761521.509911688;-0.00195 2.38388149999082e-09 -6174.59542492847 -761773.239879545;-0.0019 2.39265483200143e-09 8184.77179480059 -761754.315442547;-0.00185 2.40057806514314e-09 22541.2310040835 -761464.743324455;-0.0018 2.40764838432895e-09 36889.6814213236 -760904.626408864;-0.00175 2.4138632775081e-09 51225.0251104092 -760074.163702647;-0.0017 2.41922053655865e-09 65542.1687919871 -758973.650265249;-0.00165 2.42371825807196e-09 79836.0256530799 -757603.477103855;-0.0016 2.427354844029e-09 94101.5171544068 -755964.131034464;-0.00155 2.4301290023681e-09 108333.574834764 -754056.194508929;-0.0015 2.43203974744399e-09 122527.142111826 -751880.345408012;-0.00145 2.43308640037807e-09 136677.176078723 -749437.356800539;-0.0014 2.43326858929952e-09 150778.649295764 -746728.09666873;-0.00135 2.43258624947749e-09 164826.55157666 -743753.527599807;-0.0013 2.43103962334406e-09 178815.891768622 -740514.706443999;-0.00125 2.42862926040815e-09 192741.699525692 -737012.78393904;-0.0012 2.42535601706021e-09 206599.027074682 -733249.00430132;-0.00115 2.42122105626803e-09 220382.950973099 -729224.704783823;-0.0011 2.41622584716349e-09 234088.573858414 -724941.315201007;-0.00105 2.4103721645206e-09 247711.026188078 -720400.357420793;-0.001 2.40366208812492e-09 261245.467969642 -715603.444823859;-0.00095 2.39609800203466e-09 274687.090480388 -710552.281730409;-0.0009 2.38768259373357e-09 288031.117975841 -705248.662794639;-0.00085 2.37841885317617e-09 301272.809386572 -699694.472367103;-0.0008 2.36831007172535e-09 314407.460002673 -693891.683825212;-0.00075 2.35735984098303e-09 327430.403145324 -687842.358872106;-0.0007 2.34557205151407e-09 340337.011824836 -681548.646804134;-0.00065 2.33295089146391e-09 353122.700384601 -675012.783747228;-0.0006 2.31950084507064e-09 365782.926130355 -668237.091862409;-0.00055 2.3052266910717e-09 378313.190944174 -661223.978520742;-0.0005 2.29013350100602e-09 390709.042882633 -653975.935448002;-0.00045 2.27422663741218e-09 402966.077758563 -646495.537839381;-0.0004 2.25751175192307e-09 415079.940705835 -638785.44344453;-0.00035 2.23999478325791e-09 427046.327726628 -630848.391623276;-0.0003 2.22168195511225e-09 438860.98722061 -622687.202372337;-0.00025 2.20257977394674e-09 450519.721495521 -614304.775323394;-0.0002 2.18269502667539e-09 462018.388258588 -605704.088712863;-0.00015 2.16203477825423e-09 473352.902088262 -596888.198323744;-0.0001 2.14060636917114e-09 484519.235885749 -587860.236399914;-5e-05 2.11841741283782e-09 495513.422305822 -578623.410533257]  x2=[-0.00235 2.18790431629907e-09 -423435.883916545 -642814.215851355;-0.0023 2.12267016920573e-09 -411244.597054933 -650681.133667418;-0.00225 2.0566818475086e-09 -398907.196946177 -658316.867574984;-0.0022 1.98996279654419e-09 -386428.067009789 -665718.704634154;-0.00215 1.92253672127361e-09 -373811.641021215 -672884.015007465;-0.0021 1.85442757786035e-09 -361062.401536535 -679810.252894262;-0.00205 1.78565956515875e-09 -348184.87829983 -686494.957435201;-0.002 1.71625711611628e-09 -335183.646633789 -692935.753586591;-0.00195 1.64624488909261e-09 -322063.325814115 -699130.352964226;-0.0019 1.57564775909864e-09 -308828.577428322 -705076.554656446;-0.00185 1.50449080895849e-09 -295484.103719493 -710772.246006101;-0.0018 1.43279932039773e-09 -282034.645915594 -716215.403361176;-0.00175 1.36059876506087e-09 -268484.982544943 -721404.09279378;-0.0017 1.28791479546144e-09 -254839.927738416 -726336.470787266;-0.00165 1.21477323586775e-09 -241104.329519015 -731010.784891218;-0.0016 1.14120007312763e-09 -227283.068079382 -735425.374344093;-0.00155 1.06722144743549e-09 -213381.054047896 -739578.670663277;-0.0015 9.92863643044777e-10 -199403.226743945 -743469.198202366;-0.00145 9.18153078929328e-10 -185354.552423014 -747095.574675451;-0.0014 8.4311629939683e-10 -171240.022512195 -750456.511648236;-0.00135 7.67779964657754e-10 -157064.651836757 -753550.814995821;-0.0013 6.9217084135311e-10 -142833.476838404 -756377.385326958;-0.00125 6.16315793044386e-10 -128551.553785848 -758935.218374669;-0.0012 5.40241770669054e-10 -114223.956978345 -761223.405353051;-0.00115 4.63975802965028e-10 -99855.7769428187 -763241.133280166;-0.0011 3.87544986867484e-10 -85452.1186252198 -764987.68526689;-0.00105 3.10976477881448e-10 -71018.0995767636 -766462.440771617;-0.001 2.34297480433571e-10 -56558.8481356889 -767664.875820739;-0.00095 1.57535238206532e-10 -42079.5016051833 -768594.56319481;-0.0009 8.07170244594799e-11 -27585.2044281237 -769251.172580331;-0.00085 3.8701323379814e-12 -13081.1063592811 -769634.470687114;-0.0008 -7.29781348231086e-11 1427.63936436365 -769744.321331168;-0.00075 -1.4980047320039e-10 15935.8778545402 -769580.685483081;-0.0007 -2.26569588182836e-10 30438.4544031956 -769143.621281891;-0.00065 -3.03258204069439e-10 44930.2163139378 -768433.284014428;-0.0006 -3.79839073760135e-10 59406.0147327642 -767449.92606014;-0.00055 -4.56284988436573e-10 73860.7064774248 -766193.896801427;-0.0005 -5.32568787229274e-10 88289.1558647705 -764665.642499502;-0.00045 -6.08663366867762e-10 102686.236535437 -762865.706135843;-0.0004 -6.84541691310224e-10 117046.833275214 -760794.72721927;-0.00035 -7.6017680134929e-10 131365.843832462 -758453.441558729;-0.0003 -8.35541824190508e-10 145638.180730909 -755842.681001868;-0.00025 -9.10609983000122e-10 159858.773077217 -752963.373139481;-0.0002 -9.85354606418753e-10 174022.568362636 -749816.540975942;-0.00015 -1.05974913803761e-09 188124.534258145 -746403.302565733;-0.0001 -1.13376714583383e-09 202159.66040241 -742724.870616211;-5e-05 -1.20738233156171e-09 216122.96018194 -738782.552056731]  x3=[-0.00235 8.84227558843485e-12 -474.171530064007 -408.225123363059;-0.0023 8.86842639128461e-12 -466.392813197643 -417.090136661224;-0.00225 8.8914262844656e-12 -458.448389185534 -425.806959819857;-0.0022 8.91126709622531e-12 -450.341080643704 -434.372495793196;-0.00215 8.92794177721777e-12 -442.073768060273 -442.783701287095;-0.0021 8.94144440300823e-12 -433.649388772037 -451.037587840295;-0.00205 8.95177017617805e-12 -425.070935920843 -459.131222886203;-0.002 8.95891542802919e-12 -416.341457390142 -467.061730794827;-0.00195 8.96287761988768e-12 -407.464054722089 -474.826293894469;-0.0019 8.96365534400562e-12 -398.441882015582 -482.422153472833;-0.00185 8.96124832406134e-12 -389.278144805622 -489.846610757177;-0.0018 8.95565741525756e-12 -379.976098924407 -497.097027873182;-0.00175 8.94688460401756e-12 -370.539049344545 -504.170828782169;-0.0017 8.9349330072794e-12 -360.970349004816 -511.065500196359;-0.00165 8.91980687138849e-12 -351.273397618889 -517.778592471828;-0.0016 8.90151157058889e-12 -341.451640467417 -524.307720478856;-0.00155 8.88005360511385e-12 -331.50856717395 -530.65056444935;-0.0015 8.85544059887635e-12 -321.447710465083 -536.804870801051;-0.00145 8.82768129676029e-12 -311.272644915299 -542.768452938217;-0.0014 8.79678556151353e-12 -300.986985676938 -548.539192028509;-0.00135 8.76276437024371e-12 -290.594387195751 -554.115037755808;-0.0013 8.72562981051807e-12 -280.098541912492 -559.494009048676;-0.00125 8.68539507606887e-12 -269.503178951015 -564.674194784226;-0.0012 8.64207446210568e-12 -258.812062793328 -569.653754467132;-0.00115 8.59568336023636e-12 -248.028991942094 -574.430918883549;-0.0011 8.5462382529985e-12 -237.157797571042 -579.003990729707;-0.00105 8.49375670800328e-12 -226.202342163769 -583.371345214956;-0.001 8.43825737169374e-12 -215.166518141413 -587.531430639041;-0.00095 8.37975996271978e-12 -204.054246479703 -591.48276894342;-0.0009 8.31828526493229e-12 -192.869475315847 -595.223956236408;-0.00085 8.25385511999867e-12 -181.616178545782 -598.753663291975;-0.0008 8.18649241964261e-12 -170.298354412267 -602.07063602201;-0.00075 8.11622109751081e-12 -158.920024084324 -605.173695921897;-0.0007 8.0430661206694e-12 -147.485230228541 -608.061740489229;-0.00065 7.96705348073333e-12 -135.998035572726 -610.733743615523;-0.0006 7.88821018463162e-12 -124.462521462443 -613.188755950791;-0.00055 7.80656424501195e-12 -112.882786410927 -615.425905240841;-0.0005 7.72214467028791e-12 -101.262944642904 -617.444396637181;-0.00045 7.63498145433242e-12 -89.6071246328247 -619.243512979431;-0.0004 7.54510556582107e-12 -77.9194676380384 -620.82261505012;-0.00035 7.45254893722909e-12 -66.2041262274231 -622.181141801802;-0.0003 7.35734445348591e-12 -54.4652628059979 -623.318610556391;-0.00025 7.25952594029127e-12 -42.7070481360405 -624.234617176654;-0.0002 7.15912815209713e-12 -30.933659855235 -624.928836209801;-0.00015 7.05618675975959e-12 -19.1492809923773 -625.401021003115;-0.0001 6.95073833786517e-12 -7.35809848116446 -625.651003791588;-5e-05 6.84282035173606e-12 4.43569832740225 -625.678695757524]  x4=[-0.00235 -2.02266917733297e-12 -2895.71387002771 -4127.20568987526;-0.0023 -2.05075132400179e-12 -2817.40791556457 -4181.05207646052;-0.00225 -2.07810484849008e-12 -2738.10094948444 -4233.41295515158;-0.0022 -2.10472003222085e-12 -2657.82114917476 -4284.26972237758;-0.00215 -2.13058741894604e-12 -2576.5970376663 -4333.60430897127;-0.0021 -2.15569781810633e-12 -2494.45747349913 -4381.39918658896;-0.00205 -2.18004230809645e-12 -2411.43164046928 -4427.63737393819;-0.002 -2.20361223943504e-12 -2327.54903725988 -4472.30244281119;-0.00195 -2.22639923783771e-12 -2242.83946696045 -4515.37852392165;-0.0019 -2.24839520719244e-12 -2157.33302647795 -4556.85031254307;-0.00185 -2.26959233243606e-12 -2071.06009584354 -4596.70307394642;-0.0018 -2.28998308233089e-12 -1984.05132741867 -4634.92264863534;-0.00175 -2.30956021214059e-12 -1896.33763500447 -4671.49545737694;-0.0017 -2.32831676620417e-12 -1807.95018285818 -4706.4085060264;-0.00165 -2.34624608040727e-12 -1718.92037462069 -4739.6493901438;-0.0016 -2.36334178454992e-12 -1629.27984215895 -4771.20629940127;-0.00155 -2.37959780460986e-12 -1539.06043432729 -4801.06802177923;-0.0015 -2.39500836490055e-12 -1448.29420565173 -4829.22394754991;-0.00145 -2.40956799012332e-12 -1357.01340494113 -4855.66407304694;-0.0014 -2.42327150731263e-12 -1265.25046382933 -4880.37900421963;-0.00135 -2.43611404767408e-12 -1173.03798525238 -4903.35995997062;-0.0013 -2.44809104831425e-12 -1080.40873186482 -4924.59877527577;-0.00125 -2.45919825386182e-12 -987.395614399322 -4944.08790408512;-0.0012 -2.46943171797956e-12 -894.03167997363 -4961.820422004;-0.00115 -2.47878780476639e-12 -800.350100349081 -4977.79002875324;-0.0011 -2.48726319004922e-12 -706.384160144841 -4991.9910504076;-0.00105 -2.49485486256403e-12 -612.167245012031 -5004.4184414117;-0.001 -2.50156012502572e-12 -517.732829771976 -5015.0677863727;-0.00095 -2.50737659508646e-12 -423.114466522749 -5023.93530162903;-0.0009 -2.51230220618213e-12 -328.345772718276 -5031.01783659476;-0.00085 -2.51633520826657e-12 -233.460419224213 -5036.31287487893;-0.0008 -2.51947416843334e-12 -138.492118354849 -5039.81853517966;-0.00075 -2.52171797142484e-12 -43.4746118952799 -5041.53357195253;-0.0007 -2.52306582002855e-12 51.5583408868861 -5041.45737585314;-0.00065 -2.52351723536028e-12 146.572975236036 -5039.5899739536;-0.0006 -2.52307205703432e-12 241.535532905009 -5035.93202973292;-0.00055 -2.52173044322039e-12 336.412274149241 -5030.48484284126;-0.0005 -2.5194928705875e-12 431.169489714334 -5023.25034863819;-0.00045 -2.51636013413456e-12 525.773512812796 -5014.23111750504;-0.0004 -2.5123333469079e-12 620.190731085689 -5003.4303539317;-0.00035 -2.50741393960586e-12 714.387598544938 -4990.85189537803;-0.0003 -2.50160366007043e-12 808.330647492065 -4976.50021091046;-0.00025 -2.49490457266625e-12 901.9865004091 -4960.38039961415;-0.0002 -2.48731905754719e-12 995.321881817454 -4942.4981887813;-0.00015 -2.47884980981064e-12 1088.30363010054 -4922.85993187625;-0.0001 -2.46949983854001e-12 1180.89870928594 -4901.47260627819;-5e-05 -2.45927246573555e-12 1273.07422078292 -4878.34381080206]  x5=0.00231306500901259  V1=ones(3,3)  V2=ones(3,3)  I1=ones(3,3)  I2=ones(3,3)  nHarmo=1  Measurements=None
      settings: AttributesFormatString=\n  SourceProductName=Simscape Electrical
  MIC-MAN 60 km : powerlib/Elements/Distributed Parameters Line  Phases=3  Frequency=60  Resistance="[0.01273  0.3864]"  Inductance="[0.9337e-3  4.1264e-3]"  Capacitance=[12.74e-9 7.751e-9]  Length=60  x1=[-0.00035 2.0920446585475e-09 0 0;-0.0003 2.07809167335098e-09 0 0;-0.00025 2.06340035207799e-09 414702.847009989 -651689.739799966;-0.0002 2.04797591448504e-09 426912.524428128 -643757.501861571;-0.00015 2.03182384080135e-09 438970.521859132 -635596.539948092;-0.0001 2.01494986978179e-09 450872.555153929 -627209.753610437;-5e-05 1.99735999666791e-09 462614.395576763 -618600.122633857]  x2=[-0.00035 3.36531105125365e-09 0 0;-0.0003 3.35376361177806e-09 0 0;-0.00025 3.34102459606054e-09 424107.292912585 -620195.130414475;-0.0002 3.32709853021272e-09 435721.675552709 -612091.229315605;-0.00015 3.31199036209949e-09 447181.248356249 -603769.855117503;-0.0001 3.29570545958104e-09 458481.939791554 -595233.9643648;-5e-05 3.27824960860569e-09 469619.734776766 -586486.589818835]  x3=[-0.00035 4.73950848909624e-12 0 0;-0.0003 4.9632762771582e-12 0 0;-0.00025 5.18528063679211e-12 2939.55966283172 -2852.62256111272;-0.0002 5.40544269090609e-12 2992.80504551509 -2796.70980760672;-0.00015 5.62368421697065e-12 3044.98709881638 -2739.80339642294;-0.0001 5.83992767481075e-12 3096.08728270053 -2681.9235461383;-5e-05 6.0540962341555e-12 3146.08744151553 -2623.09082118802]  x4=[-0.00035 6.35053405942669e-13 0 0;-0.0003 3.20323945068615e-13 0 0;-0.00025 5.4806746221399e-15 -30.7557270701598 -1956.36490774189;-0.0002 -3.09364543081932e-13 6.12416964933854 -1956.5971968756;-0.00015 -6.24099845036923e-13 43.0018904805214 -1956.13431634182;-0.0001 -9.38613407288697e-13 79.8643329447751 -1954.97643059982;-5e-05 -1.25279348466618e-12 116.698399991817 -1953.12395104087]  x5=0.000339324940197445  V1=ones(3,3)  V2=ones(3,3)  I1=ones(3,3)  I2=ones(3,3)  nHarmo=1  Measurements=None
      settings: AttributesFormatString=\n  SourceProductName=Simscape Electrical
  Regulateurs6 : Subsystem
  Regulateurs7 : Subsystem
  "MIC7a " : PMIOPort  Side=Left
  MIC7b : PMIOPort  Port=2  Side=Left
  MIC7c : PMIOPort  Port=3  Side=Left
  QUE7a : PMIOPort  Port=4  Side=Left
  QUE7b : PMIOPort  Port=5  Side=Left
  QUE7c : PMIOPort  Port=6  Side=Left
  wires:
  Regulateurs6/1(Pm) -> "B_6 CHU-5600 MVA "/1
  Regulateurs6/2(Vf) -> "B_6 CHU-5600 MVA "/2
  "B_6 CHU-5600 MVA "/1 -> Regulateurs6/1(m)
  Regulateurs7/1(Pm) -> B_7 MAN 5000 MVA/1
  Regulateurs7/2(Vf) -> B_7 MAN 5000 MVA/2
  B_7 MAN 5000 MVA/1 -> Regulateurs7/1(m)
  connections:
  "Cs PER "/RConn3 -- MIC-LTD 409 km/LConn3
  "Cs PER "/RConn2 -- MIC-LTD 409 km/LConn2
  "Cs PER "/RConn1 -- MIC-LTD 409 km/LConn1
  Cs BER/RConn3 -- MAN-LEV 3*379km/LConn3
  Cs BER/RConn2 -- MAN-LEV 3*379km/LConn2
  Cs BER/RConn1 -- MAN-LEV 3*379km/LConn1
  Cs ARNS2/RConn3 -- ARN-MAN 2*169km/LConn3
  Cs ARNS2/RConn2 -- ARN-MAN 2*169km/LConn2
  Cs ARNS2/RConn1 -- ARN-MAN 2*169km/LConn1
  CHU-ARN 3*450km/RConn3 -- "Cs MTG+ARNN "/LConn3
  CHU-ARN 3*450km/RConn2 -- "Cs MTG+ARNN "/LConn2
  CHU-ARN 3*450km/RConn1 -- "Cs MTG+ARNN "/LConn1
  Load Flow Bus2/LConn1 -- 5600 MVA 13.8 kV/735 kV1/RConn3 -- CHU-ARN 3*450km/LConn3 -- CHU 330 Mvar/LConn3
  5600 MVA 13.8 kV/735 kV1/RConn2 -- CHU-ARN 3*450km/LConn2 -- CHU 330 Mvar/LConn2
  5600 MVA 13.8 kV/735 kV1/RConn1 -- CHU-ARN 3*450km/LConn1 -- CHU 330 Mvar/LConn1
  "B_6 CHU-5600 MVA "/RConn3 -- Load Flow Bus1/LConn1 -- 5600 MVA 13.8 kV/735 kV1/LConn3 -- 280 MW/LConn3
  5600 MVA 13.8 kV/735 kV1/LConn2 -- "B_6 CHU-5600 MVA "/RConn2 -- 280 MW/LConn2
  5600 MVA 13.8 kV/735 kV1/LConn1 -- "B_6 CHU-5600 MVA "/RConn1 -- 280 MW/LConn1
  "Cs ARNS1 "/RConn1 -- ARN-MIC 180km/LConn1
  "Cs ARNS1 "/RConn2 -- ARN-MIC 180km/LConn2
  "Cs ARNS1 "/RConn3 -- ARN-MIC 180km/LConn3
  "Cs PER "/LConn3 -- Load Flow Bus6/LConn1 -- MIC7c/RConn1 -- MIC-MAN 60 km/LConn3 -- ARN-MIC 180km/RConn3
  "Cs PER "/LConn2 -- MIC7b/RConn1 -- ARN-MIC 180km/RConn2 -- MIC-MAN 60 km/LConn2
  "Cs PER "/LConn1 -- "MIC7a "/RConn1 -- ARN-MIC 180km/RConn1 -- MIC-MAN 60 km/LConn1
  ARN-MAN 2*169km/RConn1 -- MAN7/LConn1
  ARN-MAN 2*169km/RConn2 -- MAN7/LConn2
  ARN-MAN 2*169km/RConn3 -- MAN7/LConn3
  Cs BER/LConn1 -- 5000 MVA 13.8 kV/735 kV2/RConn1 -- MIC-MAN 60 km/RConn1 -- MAN-MIC 1650 Mvar/LConn1 -- MAN7/RConn1
  Cs BER/LConn2 -- 5000 MVA 13.8 kV/735 kV2/RConn2 -- MIC-MAN 60 km/RConn2 -- MAN-MIC 1650 Mvar/LConn2 -- MAN7/RConn2
  Cs BER/LConn3 -- Load Flow Bus5/LConn1 -- 5000 MVA 13.8 kV/735 kV2/RConn3 -- MIC-MAN 60 km/RConn3 -- MAN-MIC 1650 Mvar/LConn3 -- MAN7/RConn3
  B_7 MAN 5000 MVA/RConn1 -- 5000 MVA 13.8 kV/735 kV2/LConn1 -- 250 MW/LConn1
  B_7 MAN 5000 MVA/RConn2 -- 5000 MVA 13.8 kV/735 kV2/LConn2 -- 250 MW/LConn2
  B_7 MAN 5000 MVA/RConn3 -- 5000 MVA 13.8 kV/735 kV2/LConn3 -- Load Flow Bus3/LConn1 -- 250 MW/LConn3
  MIC-LTD 409 km/RConn2 -- MAN-LEV 3*379km/RConn2 -- QUE7b/RConn1
  Cs ARNS2/LConn1 -- ARN 990 Mvar/LConn1 -- "Cs MTG+ARNN "/RConn1 -- "Cs ARNS1 "/LConn1
  Cs ARNS2/LConn2 -- ARN 990 Mvar/LConn2 -- "Cs MTG+ARNN "/RConn2 -- "Cs ARNS1 "/LConn2
  Cs ARNS2/LConn3 -- Load Flow Bus4/LConn1 -- "Cs ARNS1 "/LConn3 -- ARN 990 Mvar/LConn3 -- "Cs MTG+ARNN "/RConn3
  MIC-LTD 409 km/RConn1 -- QUE7a/RConn1 -- MAN-LEV 3*379km/RConn1
  MIC-LTD 409 km/RConn3 -- QUE7c/RConn1 -- MAN-LEV 3*379km/RConn3
